simulink model "control_pos_6dof_sinMI"  (R2023b)
settings: Solver=ode45  StartTime=0.0  StopTime=tsim  FixedStep=tstep  MaxStep=tstep  RelTol=tstep/10
undefined symbols (not defined in the file): a0, a1, robot_params, t_qeq_init, t_tr_init, tau_L, tr_ref
(part 5 of 7)

== matlab function control_pos_6dof_sinMI/Controlador/Controlador no lineal ==
  data: robot_params input; tau_R output size=[6,1]; q_ref input size=[6,1]; dq_ref input size=[6,1]; ddq_ref input size=[6,1]; q input size=[6,1]; dq input size=[6,1]; A0 input size=[6,1]; A1 input size=[6,1]
function tau_R = fcn(robot_params,q_ref,dq_ref,ddq_ref,q,dq,A0,A1)

% l1 = robot_params.l(1);
l2 = robot_params.l(2);
l3 = robot_params.l(3);
% l4 = robot_params.l(4);
% l5 = robot_params.l(5);
% l6 = robot_params.l(6);

% lc1 = robot_params.lc(1);
lc2 = robot_params.lc(2);
lc3 = robot_params.lc(3);
% lc4 = robot_params.lc(4);
% lc5 = robot_params.lc(5);
% lc6 = robot_params.lc(6);

d1 = robot_params.d(1);
d2 = robot_params.d(2);
d3 = robot_params.d(3);
d4 = robot_params.d(4);
d5 = robot_params.d(5);
d6 = robot_params.d(6);

% dc1 = robot_params.dc(1);
% dc2 = robot_params.dc(2);
% dc3 = robot_params.dc(3);
dc4 = robot_params.dc(4);
dc5 = robot_params.dc(5);
dc6 = robot_params.dc(6);

m1 = robot_params.m(1);
m2 = robot_params.m(2);
m3 = robot_params.m(3);
m4 = robot_params.m(4);
m5 = robot_params.m(5);
m6 = robot_params.m(6);

g = 9.81;

%Posiciones angulares
q1 = q(1);
q2 = q(2);
q3 = q(3);
q4 = q(4);
q5 = q(5);
q6 = q(6);

%Velocidades angulares
dq1 = dq(1);
dq2 = dq(2);
dq3 = dq(3);
dq4 = dq(4);
dq5 = dq(5);
dq6 = dq(6);

% Matriz de Inercia D
D = zeros(6,6);

D(1,1) = (d1*m1)/2 + (d2*m2)/2 + (d3*m3)/2 + (d4*m4)/2 + (d5*m5)/2 + (d6*m6)/2 + d4^2*m5 + d4^2*m6 + (d5^2*m6)/2 + dc4^2*m4 + (dc5^2*m5)/2 + (3*dc6^2*m6)/4 + (l2^2*m3)/2 + (l2^2*m4)/2 + (l2^2*m5)/2 + (l3^2*m4)/2 + (l2^2*m6)/2 + (l3^2*m5)/2 + (l3^2*m6)/2 + (lc2^2*m2)/2 + (lc3^2*m3)/2 - (dc6^2*m6*cos(2*q2 + 2*q3 + 2*q4 - 2*q5))/8 - (dc6^2*m6*cos(2*q2 + 2*q3 + 2*q4 + 2*q5))/8 - (d5^2*m6*cos(2*q2 + 2*q3 + 2*q4))/2 + (dc6^2*m6*cos(2*q5))/4 - (dc5^2*m5*cos(2*q2 + 2*q3 + 2*q4))/2 + (dc6^2*m6*cos(2*q2 + 2*q3 + 2*q4))/4 + (l2^2*m3*cos(2*q2))/2 + (l2^2*m4*cos(2*q2))/2 + (l2^2*m5*cos(2*q2))/2 + (l2^2*m6*cos(2*q2))/2 + (lc2^2*m2*cos(2*q2))/2 + (l3^2*m4*cos(2*q2 + 2*q3))/2 + (l3^2*m5*cos(2*q2 + 2*q3))/2 + (l3^2*m6*cos(2*q2 + 2*q3))/2 + (lc3^2*m3*cos(2*q2 + 2*q3))/2 + d5*l2*m6*sin(2*q2 + q3 + q4) + dc5*l2*m5*sin(2*q2 + q3 + q4) + (dc6*l2*m6*sin(q3 + q4 - q5))/2 + (d5*dc6*m6*cos(2*q2 + 2*q3 + 2*q4 + q5))/2 + d5*l2*m6*sin(q3 + q4) + dc5*l2*m5*sin(q3 + q4) - (dc6*l3*m6*sin(q4 + q5))/2 + (dc6*l3*m6*sin(2*q2 + 2*q3 + q4 - q5))/2 + 2*d4*dc6*m6*cos(q5) + l2*l3*m4*cos(q3) + l2*l3*m5*cos(q3) + l2*l3*m6*cos(q3) + l2*lc3*m3*cos(q3) + d5*l3*m6*sin(q4) + d5*l3*m6*sin(2*q2 + 2*q3 + q4) + dc5*l3*m5*sin(q4) + dc5*l3*m5*sin(2*q2 + 2*q3 + q4) - (dc6*l2*m6*sin(2*q2 + q3 + q4 + q5))/2 - (d5*dc6*m6*cos(2*q2 + 2*q3 + 2*q4 - q5))/2 + l2*l3*m4*cos(2*q2 + q3) + l2*l3*m5*cos(2*q2 + q3) + l2*l3*m6*cos(2*q2 + q3) + l2*lc3*m3*cos(2*q2 + q3) + (dc6*l3*m6*sin(q4 - q5))/2 - (dc6*l2*m6*sin(q3 + q4 + q5))/2 + (dc6*l2*m6*sin(2*q2 + q3 + q4 - q5))/2 - (dc6*l3*m6*sin(2*q2 + 2*q3 + q4 + q5))/2;
D(1,2) = (dc6^2*m6*cos(q2 + q3 + q4 - 2*q5))/4 - (dc6^2*m6*cos(q2 + q3 + q4 + 2*q5))/4 - (d4*dc6*m6*cos(q2 + q3 + q4 + q5))/2 + (d5*dc6*m6*cos(q2 + q3 + q4 + q5))/2 - (dc6*l3*m6*sin(q2 + q3 - q5))/2 - d4*l3*m5*sin(q2 + q3) - d4*l3*m6*sin(q2 + q3) - dc4*l3*m4*sin(q2 + q3) - (dc6*l2*m6*sin(q2 + q5))/2 + (d4*dc6*m6*cos(q2 + q3 + q4 - q5))/2 + (d5*dc6*m6*cos(q2 + q3 + q4 - q5))/2 - d4*l2*m5*sin(q2) - d4*l2*m6*sin(q2) - dc4*l2*m4*sin(q2) + d4*d5*m6*cos(q2 + q3 + q4) + d4*dc5*m5*cos(q2 + q3 + q4) - (dc6*l2*m6*sin(q2 - q5))/2 - (dc6*l3*m6*sin(q2 + q3 + q5))/2;
D(1,3) = (dc6^2*m6*cos(q2 + q3 + q4 - 2*q5))/4 - (dc6^2*m6*cos(q2 + q3 + q4 + 2*q5))/4 - (d4*dc6*m6*cos(q2 + q3 + q4 + q5))/2 + (d5*dc6*m6*cos(q2 + q3 + q4 + q5))/2 - (dc6*l3*m6*sin(q2 + q3 - q5))/2 - d4*l3*m5*sin(q2 + q3) - d4*l3*m6*sin(q2 + q3) - dc4*l3*m4*sin(q2 + q3) + (d4*dc6*m6*cos(q2 + q3 + q4 - q5))/2 + (d5*dc6*m6*cos(q2 + q3 + q4 - q5))/2 + d4*d5*m6*cos(q2 + q3 + q4) + d4*dc5*m5*cos(q2 + q3 + q4) - (dc6*l3*m6*sin(q2 + q3 + q5))/2;
D(1,4) = (dc6^2*m6*cos(q2 + q3 + q4 - 2*q5))/4 - (dc6^2*m6*cos(q2 + q3 + q4 + 2*q5))/4 - (d4*dc6*m6*cos(q2 + q3 + q4 + q5))/2 + (d5*dc6*m6*cos(q2 + q3 + q4 + q5))/2 + (d4*dc6*m6*cos(q2 + q3 + q4 - q5))/2 + (d5*dc6*m6*cos(q2 + q3 + q4 - q5))/2 + d4*d5*m6*cos(q2 + q3 + q4) + d4*dc5*m5*cos(q2 + q3 + q4);
D(1,5) = -(dc6*m6*(d4*cos(q2 + q3 + q4 + q5) + d5*cos(q2 + q3 + q4 + q5) + l3*sin(q2 + q3 - q5) - l2*sin(q2 + q5) + d4*cos(q2 + q3 + q4 - q5) - d5*cos(q2 + q3 + q4 - q5) + 2*dc6*cos(q2 + q3 + q4) + l2*sin(q2 - q5) - l3*sin(q2 + q3 + q5)))/2;
D(1,6) = 0;

D(2,1) = (dc6^2*m6*cos(q2 + q3 + q4 - 2*q5))/4 - (dc6^2*m6*cos(q2 + q3 + q4 + 2*q5))/4 - (d4*dc6*m6*cos(q2 + q3 + q4 + q5))/2 + (d5*dc6*m6*cos(q2 + q3 + q4 + q5))/2 - (dc6*l3*m6*sin(q2 + q3 - q5))/2 - d4*l3*m5*sin(q2 + q3) - d4*l3*m6*sin(q2 + q3) - dc4*l3*m4*sin(q2 + q3) - (dc6*l2*m6*sin(q2 + q5))/2 + (d4*dc6*m6*cos(q2 + q3 + q4 - q5))/2 + (d5*dc6*m6*cos(q2 + q3 + q4 - q5))/2 - d4*l2*m5*sin(q2) - d4*l2*m6*sin(q2) - dc4*l2*m4*sin(q2) + d4*d5*m6*cos(q2 + q3 + q4) + d4*dc5*m5*cos(q2 + q3 + q4) - (dc6*l2*m6*sin(q2 - q5))/2 - (dc6*l3*m6*sin(q2 + q3 + q5))/2;
D(2,2) = (d2*m2)/2 + (d3*m3)/2 + d4*m4 + (d5*m5)/2 + d5^2*m6 + dc5^2*m5 + (dc6^2*m6)/2 + l2^2*m3 + l2^2*m4 + l2^2*m5 + l3^2*m4 + l2^2*m6 + l3^2*m5 + l3^2*m6 + lc2^2*m2 + lc3^2*m3 - (dc6^2*m6*cos(2*q5))/2 + 2*d5*l2*m6*sin(q3 + q4) + 2*dc5*l2*m5*sin(q3 + q4) + 2*l2*l3*m4*cos(q3) + 2*l2*l3*m5*cos(q3) + 2*l2*l3*m6*cos(q3) + 2*l2*lc3*m3*cos(q3) + 2*d5*l3*m6*sin(q4) + 2*dc5*l3*m5*sin(q4) - 2*dc6*l3*m6*cos(q4)*sin(q5) - 2*dc6*l2*m6*cos(q3)*cos(q4)*sin(q5) + 2*dc6*l2*m6*sin(q3)*sin(q4)*sin(q5);
D(2,3) = d5^2*m6 + dc5^2*m5 + (dc6^2*m6)/2 + l3^2*m4 + l3^2*m5 + l3^2*m6 + lc3^2*m3 - (dc6^2*m6*cos(2*q5))/2 + d5*l2*m6*sin(q3 + q4) + dc5*l2*m5*sin(q3 + q4) + l2*l3*m4*cos(q3) + l2*l3*m5*cos(q3) + l2*l3*m6*cos(q3) + l2*lc3*m3*cos(q3) + 2*d5*l3*m6*sin(q4) + 2*dc5*l3*m5*sin(q4) - 2*dc6*l3*m6*cos(q4)*sin(q5) - dc6*l2*m6*cos(q3)*cos(q4)*sin(q5) + dc6*l2*m6*sin(q3)*sin(q4)*sin(q5);
D(2,4) = d5^2*m6 + dc5^2*m5 + (dc6^2*m6)/2 - (dc6^2*m6*cos(2*q5))/2 + d5*l2*m6*sin(q3 + q4) + dc5*l2*m5*sin(q3 + q4) + d5*l3*m6*sin(q4) + dc5*l3*m5*sin(q4) - dc6*l3*m6*cos(q4)*sin(q5) - dc6*l2*m6*cos(q3)*cos(q4)*sin(q5) + dc6*l2*m6*sin(q3)*sin(q4)*sin(q5);
D(2,5) = -dc6*m6*cos(q5)*(d5 + l2*sin(q3 + q4) + l3*sin(q4));
D(2,6) = 0;

D(3,1) = (dc6^2*m6*cos(q2 + q3 + q4 - 2*q5))/4 - (dc6^2*m6*cos(q2 + q3 + q4 + 2*q5))/4 - (d4*dc6*m6*cos(q2 + q3 + q4 + q5))/2 + (d5*dc6*m6*cos(q2 + q3 + q4 + q5))/2 - (dc6*l3*m6*sin(q2 + q3 - q5))/2 - d4*l3*m5*sin(q2 + q3) - d4*l3*m6*sin(q2 + q3) - dc4*l3*m4*sin(q2 + q3) + (d4*dc6*m6*cos(q2 + q3 + q4 - q5))/2 + (d5*dc6*m6*cos(q2 + q3 + q4 - q5))/2 + d4*d5*m6*cos(q2 + q3 + q4) + d4*dc5*m5*cos(q2 + q3 + q4) - (dc6*l3*m6*sin(q2 + q3 + q5))/2;
D(3,2) = d5^2*m6 + dc5^2*m5 + (dc6^2*m6)/2 + l3^2*m4 + l3^2*m5 + l3^2*m6 + lc3^2*m3 - (dc6^2*m6*cos(2*q5))/2 + d5*l2*m6*sin(q3 + q4) + dc5*l2*m5*sin(q3 + q4) + l2*l3*m4*cos(q3) + l2*l3*m5*cos(q3) + l2*l3*m6*cos(q3) + l2*lc3*m3*cos(q3) + 2*d5*l3*m6*sin(q4) + 2*dc5*l3*m5*sin(q4) - 2*dc6*l3*m6*cos(q4)*sin(q5) - dc6*l2*m6*cos(q3)*cos(q4)*sin(q5) + dc6*l2*m6*sin(q3)*sin(q4)*sin(q5);
D(3,3) = (d3*m3)/2 + d4*m4 + (d5*m5)/2 + d5^2*m6 + dc5^2*m5 + l3^2*m4 + l3^2*m5 + l3^2*m6 + lc3^2*m3 + dc6^2*m6*sin(q5)^2 + 2*d5*l3*m6*sin(q4) + 2*dc5*l3*m5*sin(q4) - 2*dc6*l3*m6*cos(q4)*sin(q5);
D(3,4) = d5^2*m6 + dc5^2*m5 + dc6^2*m6*sin(q5)^2 + d5*l3*m6*sin(q4) + dc5*l3*m5*sin(q4) - dc6*l3*m6*cos(q4)*sin(q5);
D(3,5) = -dc6*m6*cos(q5)*(d5 + l3*sin(q4));
D(3,6) = 0;

D(4,1) = (dc6^2*m6*cos(q2 + q3 + q4 - 2*q5))/4 - (dc6^2*m6*cos(q2 + q3 + q4 + 2*q5))/4 - (d4*dc6*m6*cos(q2 + q3 + q4 + q5))/2 + (d5*dc6*m6*cos(q2 + q3 + q4 + q5))/2 + (d4*dc6*m6*cos(q2 + q3 + q4 - q5))/2 + (d5*dc6*m6*cos(q2 + q3 + q4 - q5))/2 + d4*d5*m6*cos(q2 + q3 + q4) + d4*dc5*m5*cos(q2 + q3 + q4);
D(4,2) = d5^2*m6 + dc5^2*m5 + (dc6^2*m6)/2 - (dc6^2*m6*cos(2*q5))/2 + d5*l2*m6*sin(q3 + q4) + dc5*l2*m5*sin(q3 + q4) + d5*l3*m6*sin(q4) + dc5*l3*m5*sin(q4) - dc6*l3*m6*cos(q4)*sin(q5) - dc6*l2*m6*cos(q3)*cos(q4)*sin(q5) + dc6*l2*m6*sin(q3)*sin(q4)*sin(q5);
D(4,3) = d5^2*m6 + dc5^2*m5 + dc6^2*m6*sin(q5)^2 + d5*l3*m6*sin(q4) + dc5*l3*m5*sin(q4) - dc6*l3*m6*cos(q4)*sin(q5);
D(4,4) = d4*m4 + (d5*m5)/2 + d5^2*m6 + dc5^2*m5 + dc6^2*m6 - dc6^2*m6*cos(q5)^2;
D(4,5) = -d5*dc6*m6*cos(q5);
D(4,6) = 0;

D(5,1) = -(dc6*m6*(d4*cos(q2 + q3 + q4 + q5) + d5*cos(q2 + q3 + q4 + q5) + l3*sin(q2 + q3 - q5) - l2*sin(q2 + q5) + d4*cos(q2 + q3 + q4 - q5) - d5*cos(q2 + q3 + q4 - q5) + 2*dc6*cos(q2 + q3 + q4) + l2*sin(q2 - q5) - l3*sin(q2 + q3 + q5)))/2;
D(5,2) = -dc6*m6*cos(q5)*(d5 + l2*sin(q3 + q4) + l3*sin(q4));
D(5,3) = -dc6*m6*cos(q5)*(d5 + l3*sin(q4));
D(5,4) = -d5*dc6*m6*cos(q5);
D(5,5) = (d4*m4)/2 + (d5*m5)/2 + dc6^2*m6;
D(5,6) = 0;

D(6,1) = 0;
D(6,2) = 0;
D(6,3) = 0;
D(6,4) = 0;
D(6,5) = 0;
D(6,6) = 1;

% Matriz de Coriollis C
C = zeros(6,6);

C(1,1) = 0;
C(1,2) = (dc6^2*dq1*m6*sin(2*q2 + 2*q3 + 2*q4 - 2*q5))/4 + (dc6^2*dq1*m6*sin(2*q2 + 2*q3 + 2*q4 + 2*q5))/4 + d5^2*dq1*m6*sin(2*q2 + 2*q3 + 2*q4) + dc5^2*dq1*m5*sin(2*q2 + 2*q3 + 2*q4) - (dc6^2*dq1*m6*sin(2*q2 + 2*q3 + 2*q4))/2 - dq1*l2^2*m3*sin(2*q2) - dq1*l2^2*m4*sin(2*q2) - dq1*l2^2*m5*sin(2*q2) - dq1*l2^2*m6*sin(2*q2) - dq1*lc2^2*m2*sin(2*q2) - dq1*l3^2*m4*sin(2*q2 + 2*q3) - dq1*l3^2*m5*sin(2*q2 + 2*q3) - dq1*l3^2*m6*sin(2*q2 + 2*q3) - dq1*lc3^2*m3*sin(2*q2 + 2*q3) - (dc6^2*dq2*m6*sin(q2 + q3 + q4 - 2*q5))/4 + (dc6^2*dq2*m6*sin(q2 + q3 + q4 + 2*q5))/4 - (dc6*dq2*l2*m6*cos(q2 - q5))/2 + d5*dc6*dq1*m6*sin(2*q2 + 2*q3 + 2*q4 - q5) - (dc6*dq2*l3*m6*cos(q2 + q3 + q5))/2 - 2*dq1*l2*l3*m4*sin(2*q2 + q3) - 2*dq1*l2*l3*m5*sin(2*q2 + q3) - 2*dq1*l2*l3*m6*sin(2*q2 + q3) - 2*dq1*l2*lc3*m3*sin(2*q2 + q3) - d4*d5*dq2*m6*sin(q2 + q3 + q4) - d4*dc5*dq2*m5*sin(q2 + q3 + q4) + dc6*dq1*l2*m6*cos(2*q2 + q3 + q4 - q5) - dc6*dq1*l3*m6*cos(2*q2 + 2*q3 + q4 + q5) + 2*d5*dq1*l2*m6*cos(2*q2 + q3 + q4) + 2*dc5*dq1*l2*m5*cos(2*q2 + q3 + q4) - (dc6*dq2*l3*m6*cos(q2 + q3 - q5))/2 + (d4*dc6*dq2*m6*sin(q2 + q3 + q4 + q5))/2 - (d5*dc6*dq2*m6*sin(q2 + q3 + q4 + q5))/2 - d4*dq2*l3*m5*cos(q2 + q3) - d4*dq2*l3*m6*cos(q2 + q3) - dc4*dq2*l3*m4*cos(q2 + q3) - (dc6*dq2*l2*m6*cos(q2 + q5))/2 + dc6*dq1*l3*m6*cos(2*q2 + 2*q3 + q4 - q5) - d5*dc6*dq1*m6*sin(2*q2 + 2*q3 + 2*q4 + q5) - d4*dq2*l2*m5*cos(q2) - d4*dq2*l2*m6*cos(q2) + 2*d5*dq1*l3*m6*cos(2*q2 + 2*q3 + q4) - dc4*dq2*l2*m4*cos(q2) + 2*dc5*dq1*l3*m5*cos(2*q2 + 2*q3 + q4) - dc6*dq1*l2*m6*cos(2*q2 + q3 + q4 + q5) - (d4*dc6*dq2*m6*sin(q2 + q3 + q4 - q5))/2 - (d5*dc6*dq2*m6*sin(q2 + q3 + q4 - q5))/2;
C(1,3) = (dc6^2*dq1*m6*sin(2*q2 + 2*q3 + 2*q4 - 2*q5))/4 + (dc6^2*dq1*m6*sin(2*q2 + 2*q3 + 2*q4 + 2*q5))/4 + d5^2*dq1*m6*sin(2*q2 + 2*q3 + 2*q4) + dc5^2*dq1*m5*sin(2*q2 + 2*q3 + 2*q4) - (dc6^2*dq1*m6*sin(2*q2 + 2*q3 + 2*q4))/2 - dq1*l3^2*m4*sin(2*q2 + 2*q3) - dq1*l3^2*m5*sin(2*q2 + 2*q3) - dq1*l3^2*m6*sin(2*q2 + 2*q3) - dq1*lc3^2*m3*sin(2*q2 + 2*q3) - (dc6^2*dq2*m6*sin(q2 + q3 + q4 - 2*q5))/2 + (dc6^2*dq2*m6*sin(q2 + q3 + q4 + 2*q5))/2 - (dc6^2*dq3*m6*sin(q2 + q3 + q4 - 2*q5))/4 + (dc6^2*dq3*m6*sin(q2 + q3 + q4 + 2*q5))/4 + d5*dc6*dq1*m6*sin(2*q2 + 2*q3 + 2*q4 - q5) - (dc6*dq1*l2*m6*cos(q3 + q4 + q5))/2 - dc6*dq2*l3*m6*cos(q2 + q3 + q5) - (dc6*dq3*l3*m6*cos(q2 + q3 + q5))/2 - dq1*l2*l3*m4*sin(2*q2 + q3) - dq1*l2*l3*m5*sin(2*q2 + q3) - dq1*l2*l3*m6*sin(2*q2 + q3) - dq1*l2*lc3*m3*sin(2*q2 + q3) - 2*d4*d5*dq2*m6*sin(q2 + q3 + q4) - d4*d5*dq3*m6*sin(q2 + q3 + q4) - 2*d4*dc5*dq2*m5*sin(q2 + q3 + q4) - d4*dc5*dq3*m5*sin(q2 + q3 + q4) + (dc6*dq1*l2*m6*cos(2*q2 + q3 + q4 - q5))/2 - dc6*dq1*l3*m6*cos(2*q2 + 2*q3 + q4 + q5) + d5*dq1*l2*m6*cos(2*q2 + q3 + q4) + dc5*dq1*l2*m5*cos(2*q2 + q3 + q4) + (dc6*dq1*l2*m6*cos(q3 + q4 - q5))/2 - dc6*dq2*l3*m6*cos(q2 + q3 - q5) - (dc6*dq3*l3*m6*cos(q2 + q3 - q5))/2 + d4*dc6*dq2*m6*sin(q2 + q3 + q4 + q5) + (d4*dc6*dq3*m6*sin(q2 + q3 + q4 + q5))/2 - d5*dc6*dq2*m6*sin(q2 + q3 + q4 + q5) - (d5*dc6*dq3*m6*sin(q2 + q3 + q4 + q5))/2 - 2*d4*dq2*l3*m5*cos(q2 + q3) - 2*d4*dq2*l3*m6*cos(q2 + q3) - d4*dq3*l3*m5*cos(q2 + q3) - d4*dq3*l3*m6*cos(q2 + q3) + d5*dq1*l2*m6*cos(q3 + q4) - 2*dc4*dq2*l3*m4*cos(q2 + q3) - dc4*dq3*l3*m4*cos(q2 + q3) + dc5*dq1*l2*m5*cos(q3 + q4) + dc6*dq1*l3*m6*cos(2*q2 + 2*q3 + q4 - q5) - d5*dc6*dq1*m6*sin(2*q2 + 2*q3 + 2*q4 + q5) + 2*d5*dq1*l3*m6*cos(2*q2 + 2*q3 + q4) + 2*dc5*dq1*l3*m5*cos(2*q2 + 2*q3 + q4) - (dc6*dq1*l2*m6*cos(2*q2 + q3 + q4 + q5))/2 - dq1*l2*l3*m4*sin(q3) - dq1*l2*l3*m5*sin(q3) - dq1*l2*l3*m6*sin(q3) - dq1*l2*lc3*m3*sin(q3) - d4*dc6*dq2*m6*sin(q2 + q3 + q4 - q5) - (d4*dc6*dq3*m6*sin(q2 + q3 + q4 - q5))/2 - d5*dc6*dq2*m6*sin(q2 + q3 + q4 - q5) - (d5*dc6*dq3*m6*sin(q2 + q3 + q4 - q5))/2;
C(1,4) = (dc6^2*dq1*m6*sin(2*q2 + 2*q3 + 2*q4 - 2*q5))/4 + (dc6^2*dq1*m6*sin(2*q2 + 2*q3 + 2*q4 + 2*q5))/4 + d5^2*dq1*m6*sin(2*q2 + 2*q3 + 2*q4) + dc5^2*dq1*m5*sin(2*q2 + 2*q3 + 2*q4) - (dc6^2*dq1*m6*sin(2*q2 + 2*q3 + 2*q4))/2 - (dc6^2*dq2*m6*sin(q2 + q3 + q4 - 2*q5))/2 + (dc6^2*dq2*m6*sin(q2 + q3 + q4 + 2*q5))/2 - (dc6^2*dq3*m6*sin(q2 + q3 + q4 - 2*q5))/2 + (dc6^2*dq3*m6*sin(q2 + q3 + q4 + 2*q5))/2 - (dc6^2*dq4*m6*sin(q2 + q3 + q4 - 2*q5))/4 + (dc6^2*dq4*m6*sin(q2 + q3 + q4 + 2*q5))/4 + (dc6*dq1*l3*m6*cos(q4 - q5))/2 + d5*dc6*dq1*m6*sin(2*q2 + 2*q3 + 2*q4 - q5) - (dc6*dq1*l2*m6*cos(q3 + q4 + q5))/2 - 2*d4*d5*dq2*m6*sin(q2 + q3 + q4) - 2*d4*d5*dq3*m6*sin(q2 + q3 + q4) - d4*d5*dq4*m6*sin(q2 + q3 + q4) - 2*d4*dc5*dq2*m5*sin(q2 + q3 + q4) - 2*d4*dc5*dq3*m5*sin(q2 + q3 + q4) - d4*dc5*dq4*m5*sin(q2 + q3 + q4) + (dc6*dq1*l2*m6*cos(2*q2 + q3 + q4 - q5))/2 - (dc6*dq1*l3*m6*cos(2*q2 + 2*q3 + q4 + q5))/2 + d5*dq1*l2*m6*cos(2*q2 + q3 + q4) + dc5*dq1*l2*m5*cos(2*q2 + q3 + q4) + (dc6*dq1*l2*m6*cos(q3 + q4 - q5))/2 + d4*dc6*dq2*m6*sin(q2 + q3 + q4 + q5) + d4*dc6*dq3*m6*sin(q2 + q3 + q4 + q5) - d5*dc6*dq2*m6*sin(q2 + q3 + q4 + q5) + (d4*dc6*dq4*m6*sin(q2 + q3 + q4 + q5))/2 - d5*dc6*dq3*m6*sin(q2 + q3 + q4 + q5) - (d5*dc6*dq4*m6*sin(q2 + q3 + q4 + q5))/2 + d5*dq1*l2*m6*cos(q3 + q4) + dc5*dq1*l2*m5*cos(q3 + q4) - (dc6*dq1*l3*m6*cos(q4 + q5))/2 + (dc6*dq1*l3*m6*cos(2*q2 + 2*q3 + q4 - q5))/2 - d5*dc6*dq1*m6*sin(2*q2 + 2*q3 + 2*q4 + q5) + d5*dq1*l3*m6*cos(q4) + d5*dq1*l3*m6*cos(2*q2 + 2*q3 + q4) + dc5*dq1*l3*m5*cos(q4) + dc5*dq1*l3*m5*cos(2*q2 + 2*q3 + q4) - (dc6*dq1*l2*m6*cos(2*q2 + q3 + q4 + q5))/2 - d4*dc6*dq2*m6*sin(q2 + q3 + q4 - q5) - d4*dc6*dq3*m6*sin(q2 + q3 + q4 - q5) - d5*dc6*dq2*m6*sin(q2 + q3 + q4 - q5) - (d4*dc6*dq4*m6*sin(q2 + q3 + q4 - q5))/2 - d5*dc6*dq3*m6*sin(q2 + q3 + q4 - q5) - (d5*dc6*dq4*m6*sin(q2 + q3 + q4 - q5))/2;
C(1,5) = (dc6*m6*(4*d4*dq2*sin(q2 + q3 + q4 - q5) - 2*dq1*l2*cos(2*q2 + q3 + q4 + q5) - 8*d4*dq1*sin(q5) + 4*d4*dq3*sin(q2 + q3 + q4 - q5) + 4*d4*dq4*sin(q2 + q3 + q4 - q5) - 2*d4*dq5*sin(q2 + q3 + q4 - q5) + 2*d5*dq5*sin(q2 + q3 + q4 - q5) + 2*dc6*dq2*sin(q2 + q3 + q4 - 2*q5) + 2*dc6*dq2*sin(q2 + q3 + q4 + 2*q5) + 2*dc6*dq3*sin(q2 + q3 + q4 - 2*q5) + 2*dc6*dq3*sin(q2 + q3 + q4 + 2*q5) + 2*dc6*dq4*sin(q2 + q3 + q4 - 2*q5) + 2*dc6*dq4*sin(q2 + q3 + q4 + 2*q5) - 2*dq1*l3*cos(q4 - q5) + 2*dq5*l2*cos(q2 - q5) - 2*d5*dq1*sin(2*q2 + 2*q3 + 2*q4 - q5) - dc6*dq1*sin(2*q2 + 2*q3 + 2*q4 - 2*q5) + dc6*dq1*sin(2*q2 + 2*q3 + 2*q4 + 2*q5) - 2*dq1*l2*cos(q3 + q4 + q5) + 2*dq5*l3*cos(q2 + q3 + q5) + 4*dc6*dq2*sin(q2 + q3 + q4) + 4*dc6*dq3*sin(q2 + q3 + q4) + 4*dc6*dq4*sin(q2 + q3 + q4) - 2*dc6*dq1*sin(2*q5) - 2*dq1*l2*cos(2*q2 + q3 + q4 - q5) - 2*dq1*l3*cos(2*q2 + 2*q3 + q4 + q5) - 2*dq1*l2*cos(q3 + q4 - q5) + 2*dq5*l3*cos(q2 + q3 - q5) + 4*d4*dq2*sin(q2 + q3 + q4 + q5) + 4*d4*dq3*sin(q2 + q3 + q4 + q5) + 4*d4*dq4*sin(q2 + q3 + q4 + q5) + 2*d4*dq5*sin(q2 + q3 + q4 + q5) + 2*d5*dq5*sin(q2 + q3 + q4 + q5) - 2*dq1*l3*cos(q4 + q5) + 2*dq5*l2*cos(q2 + q5) - 2*dq1*l3*cos(2*q2 + 2*q3 + q4 - q5) - 2*d5*dq1*sin(2*q2 + 2*q3 + 2*q4 + q5)))/4;
C(1,6) = 0;

C(2,1) = (dc6^2*dq1*m6*sin(2*q2 + 2*q3 + 2*q4))/4 - (dc6^2*dq1*m6*sin(2*q2 + 2*q3 + 2*q4 + 2*q5))/8 - (d5^2*dq1*m6*sin(2*q2 + 2*q3 + 2*q4))/2 - (dc5^2*dq1*m5*sin(2*q2 + 2*q3 + 2*q4))/2 - (dc6^2*dq1*m6*sin(2*q2 + 2*q3 + 2*q4 - 2*q5))/8 + (dq1*l2^2*m3*sin(2*q2))/2 + (dq1*l2^2*m4*sin(2*q2))/2 + (dq1*l2^2*m5*sin(2*q2))/2 + (dq1*l2^2*m6*sin(2*q2))/2 + (dq1*lc2^2*m2*sin(2*q2))/2 + (dq1*l3^2*m4*sin(2*q2 + 2*q3))/2 + (dq1*l3^2*m5*sin(2*q2 + 2*q3))/2 + (dq1*l3^2*m6*sin(2*q2 + 2*q3))/2 + (dq1*lc3^2*m3*sin(2*q2 + 2*q3))/2 - (d5*dc6*dq1*m6*sin(2*q2 + 2*q3 + 2*q4 - q5))/2 + dq1*l2*l3*m4*sin(2*q2 + q3) + dq1*l2*l3*m5*sin(2*q2 + q3) + dq1*l2*l3*m6*sin(2*q2 + q3) + dq1*l2*lc3*m3*sin(2*q2 + q3) - (dc6*dq1*l2*m6*cos(2*q2 + q3 + q4 - q5))/2 + (dc6*dq1*l3*m6*cos(2*q2 + 2*q3 + q4 + q5))/2 - d5*dq1*l2*m6*cos(2*q2 + q3 + q4) - dc5*dq1*l2*m5*cos(2*q2 + q3 + q4) - (dc6*dq1*l3*m6*cos(2*q2 + 2*q3 + q4 - q5))/2 + (d5*dc6*dq1*m6*sin(2*q2 + 2*q3 + 2*q4 + q5))/2 - d5*dq1*l3*m6*cos(2*q2 + 2*q3 + q4) - dc5*dq1*l3*m5*cos(2*q2 + 2*q3 + q4) + (dc6*dq1*l2*m6*cos(2*q2 + q3 + q4 + q5))/2;
C(2,2) = 0;
C(2,3) = -l2*(2*dq2 + dq3)*(l3*m4*sin(q3) + l3*m5*sin(q3) + l3*m6*sin(q3) + lc3*m3*sin(q3) - d5*m6*cos(q3 + q4) - dc5*m5*cos(q3 + q4) - dc6*m6*cos(q3)*sin(q4)*sin(q5) - dc6*m6*cos(q4)*sin(q3)*sin(q5));
C(2,4) = (dc6*dq4*l3*m6*cos(q4 - q5))/2 + 2*d5*dq2*l2*m6*cos(q3 + q4) + 2*d5*dq3*l2*m6*cos(q3 + q4) + d5*dq4*l2*m6*cos(q3 + q4) + 2*dc5*dq2*l2*m5*cos(q3 + q4) + 2*dc5*dq3*l2*m5*cos(q3 + q4) + dc5*dq4*l2*m5*cos(q3 + q4) - (dc6*dq4*l3*m6*cos(q4 + q5))/2 + 2*d5*dq2*l3*m6*cos(q4) + 2*d5*dq3*l3*m6*cos(q4) + d5*dq4*l3*m6*cos(q4) + 2*dc5*dq2*l3*m5*cos(q4) + 2*dc5*dq3*l3*m5*cos(q4) + dc5*dq4*l3*m5*cos(q4) + 2*dc6*dq2*l3*m6*sin(q4)*sin(q5) + 2*dc6*dq3*l3*m6*sin(q4)*sin(q5) + 2*dc6*dq2*l2*m6*cos(q3)*sin(q4)*sin(q5) + 2*dc6*dq2*l2*m6*cos(q4)*sin(q3)*sin(q5) + 2*dc6*dq3*l2*m6*cos(q3)*sin(q4)*sin(q5) + 2*dc6*dq3*l2*m6*cos(q4)*sin(q3)*sin(q5) + dc6*dq4*l2*m6*cos(q3)*sin(q4)*sin(q5) + dc6*dq4*l2*m6*cos(q4)*sin(q3)*sin(q5);
C(2,5) = -(dc6*m6*(2*dq2*l3*cos(q4 - q5) - 2*d5*dq1*sin(q2 + q3 + q4 - q5) - dc6*dq1*sin(q2 + q3 + q4 - 2*q5) - dc6*dq1*sin(q2 + q3 + q4 + 2*q5) - 2*dq1*l2*cos(q2 - q5) - 2*d5*dq5*sin(q5) + 2*dq3*l3*cos(q4 - q5) + 2*dq4*l3*cos(q4 - q5) - dq5*l3*cos(q4 - q5) + 2*dq1*l3*cos(q2 + q3 + q5) + 2*dq2*l2*cos(q3 + q4 + q5) + 2*dq3*l2*cos(q3 + q4 + q5) + 2*dq4*l2*cos(q3 + q4 + q5) + dq5*l2*cos(q3 + q4 + q5) + 2*dc6*dq1*sin(q2 + q3 + q4) - 2*dc6*dq2*sin(2*q5) - 2*dc6*dq3*sin(2*q5) - 2*dc6*dq4*sin(2*q5) - 2*dq1*l3*cos(q2 + q3 - q5) + 2*dq2*l2*cos(q3 + q4 - q5) + 2*dq3*l2*cos(q3 + q4 - q5) + 2*dq4*l2*cos(q3 + q4 - q5) - dq5*l2*cos(q3 + q4 - q5) + 2*d5*dq1*sin(q2 + q3 + q4 + q5) + 2*dq1*l2*cos(q2 + q5) + 2*dq2*l3*cos(q4 + q5) + 2*dq3*l3*cos(q4 + q5) + 2*dq4*l3*cos(q4 + q5) + dq5*l3*cos(q4 + q5)))/2;
C(2,6) = 0;

C(3,1) = (dc6^2*dq1*m6*sin(2*q2 + 2*q3 + 2*q4))/4 - (dc6^2*dq1*m6*sin(2*q2 + 2*q3 + 2*q4 + 2*q5))/8 - (d5^2*dq1*m6*sin(2*q2 + 2*q3 + 2*q4))/2 - (dc5^2*dq1*m5*sin(2*q2 + 2*q3 + 2*q4))/2 - (dc6^2*dq1*m6*sin(2*q2 + 2*q3 + 2*q4 - 2*q5))/8 + (dq1*l3^2*m4*sin(2*q2 + 2*q3))/2 + (dq1*l3^2*m5*sin(2*q2 + 2*q3))/2 + (dq1*l3^2*m6*sin(2*q2 + 2*q3))/2 + (dq1*lc3^2*m3*sin(2*q2 + 2*q3))/2 - (d5*dc6*dq1*m6*sin(2*q2 + 2*q3 + 2*q4 - q5))/2 + (dc6*dq1*l2*m6*cos(q3 + q4 + q5))/4 + (dq1*l2*l3*m4*sin(2*q2 + q3))/2 + (dq1*l2*l3*m5*sin(2*q2 + q3))/2 + (dq1*l2*l3*m6*sin(2*q2 + q3))/2 + (dq1*l2*lc3*m3*sin(2*q2 + q3))/2 - (dc6*dq1*l2*m6*cos(2*q2 + q3 + q4 - q5))/4 + (dc6*dq1*l3*m6*cos(2*q2 + 2*q3 + q4 + q5))/2 - (d5*dq1*l2*m6*cos(2*q2 + q3 + q4))/2 - (dc5*dq1*l2*m5*cos(2*q2 + q3 + q4))/2 - (dc6*dq1*l2*m6*cos(q3 + q4 - q5))/4 - (d5*dq1*l2*m6*cos(q3 + q4))/2 - (dc5*dq1*l2*m5*cos(q3 + q4))/2 - (dc6*dq1*l3*m6*cos(2*q2 + 2*q3 + q4 - q5))/2 + (d5*dc6*dq1*m6*sin(2*q2 + 2*q3 + 2*q4 + q5))/2 - d5*dq1*l3*m6*cos(2*q2 + 2*q3 + q4) - dc5*dq1*l3*m5*cos(2*q2 + 2*q3 + q4) + (dc6*dq1*l2*m6*cos(2*q2 + q3 + q4 + q5))/4 + (dq1*l2*l3*m4*sin(q3))/2 + (dq1*l2*l3*m5*sin(q3))/2 + (dq1*l2*l3*m6*sin(q3))/2 + (dq1*l2*lc3*m3*sin(q3))/2;
C(3,2) = dq2*l2*(l3*m4*sin(q3) + l3*m5*sin(q3) + l3*m6*sin(q3) + lc3*m3*sin(q3) - d5*m6*cos(q3 + q4) - dc5*m5*cos(q3 + q4) - dc6*m6*cos(q3)*sin(q4)*sin(q5) - dc6*m6*cos(q4)*sin(q3)*sin(q5));
C(3,3) = 0;
C(3,4) = l3*(2*dq2 + 2*dq3 + dq4)*(d5*m6*cos(q4) + dc5*m5*cos(q4) + dc6*m6*sin(q4)*sin(q5));
C(3,5) = -dc6*m6*(dq2*l3*cos(q4 - q5) - d5*dq1*sin(q2 + q3 + q4 - q5) - (dc6*dq1*sin(q2 + q3 + q4 - 2*q5))/2 - (dc6*dq1*sin(q2 + q3 + q4 + 2*q5))/2 - d5*dq5*sin(q5) + dq3*l3*cos(q4 - q5) + dq4*l3*cos(q4 - q5) - (dq5*l3*cos(q4 - q5))/2 + dq1*l3*cos(q2 + q3 + q5) + dc6*dq1*sin(q2 + q3 + q4) - dc6*dq2*sin(2*q5) - dc6*dq3*sin(2*q5) - dc6*dq4*sin(2*q5) - dq1*l3*cos(q2 + q3 - q5) + d5*dq1*sin(q2 + q3 + q4 + q5) + dq2*l3*cos(q4 + q5) + dq3*l3*cos(q4 + q5) + dq4*l3*cos(q4 + q5) + (dq5*l3*cos(q4 + q5))/2);
C(3,6) = 0;

C(4,1) = (dc6^2*dq1*m6*sin(2*q2 + 2*q3 + 2*q4))/4 - (dc6^2*dq1*m6*sin(2*q2 + 2*q3 + 2*q4 + 2*q5))/8 - (d5^2*dq1*m6*sin(2*q2 + 2*q3 + 2*q4))/2 - (dc5^2*dq1*m5*sin(2*q2 + 2*q3 + 2*q4))/2 - (dc6^2*dq1*m6*sin(2*q2 + 2*q3 + 2*q4 - 2*q5))/8 - (dc6*dq1*l3*m6*cos(q4 - q5))/4 - (d5*dc6*dq1*m6*sin(2*q2 + 2*q3 + 2*q4 - q5))/2 + (dc6*dq1*l2*m6*cos(q3 + q4 + q5))/4 - (dc6*dq1*l2*m6*cos(2*q2 + q3 + q4 - q5))/4 + (dc6*dq1*l3*m6*cos(2*q2 + 2*q3 + q4 + q5))/4 - (d5*dq1*l2*m6*cos(2*q2 + q3 + q4))/2 - (dc5*dq1*l2*m5*cos(2*q2 + q3 + q4))/2 - (dc6*dq1*l2*m6*cos(q3 + q4 - q5))/4 - (d5*dq1*l2*m6*cos(q3 + q4))/2 - (dc5*dq1*l2*m5*cos(q3 + q4))/2 + (dc6*dq1*l3*m6*cos(q4 + q5))/4 - (dc6*dq1*l3*m6*cos(2*q2 + 2*q3 + q4 - q5))/4 + (d5*dc6*dq1*m6*sin(2*q2 + 2*q3 + 2*q4 + q5))/2 - (d5*dq1*l3*m6*cos(q4))/2 - (d5*dq1*l3*m6*cos(2*q2 + 2*q3 + q4))/2 - (dc5*dq1*l3*m5*cos(q4))/2 - (dc5*dq1*l3*m5*cos(2*q2 + 2*q3 + q4))/2 + (dc6*dq1*l2*m6*cos(2*q2 + q3 + q4 + q5))/4;
C(4,2) = - dq2*(l2*cos(q3 + q4) + l3*cos(q4))*(d5*m6 + dc5*m5) - dc6*dq2*l3*m6*sin(q4)*sin(q5) - dc6*dq2*l2*m6*cos(q3)*sin(q4)*sin(q5) - dc6*dq2*l2*m6*cos(q4)*sin(q3)*sin(q5);
C(4,3) = -l3*(2*dq2 + dq3)*(d5*m6*cos(q4) + dc5*m5*cos(q4) + dc6*m6*sin(q4)*sin(q5));
C(4,4) = 0;
C(4,5) = (dc6*m6*(2*d5*dq5*sin(q5) + 2*d5*dq1*sin(q2 + q3 + q4 - q5) + dc6*dq1*sin(q2 + q3 + q4 - 2*q5) + dc6*dq1*sin(q2 + q3 + q4 + 2*q5) - 2*dc6*dq1*sin(q2 + q3 + q4) + 2*dc6*dq2*sin(2*q5) + 2*dc6*dq3*sin(2*q5) + 2*dc6*dq4*sin(2*q5) - 2*d5*dq1*sin(q2 + q3 + q4 + q5)))/2;
C(4,6) = 0;

C(5,1) = (dc6*dq1*m6*(2*dc6*sin(2*q5) + 2*l2*cos(2*q2 + q3 + q4 - q5) + 2*l3*cos(2*q2 + 2*q3 + q4 + q5) + 2*l2*cos(q3 + q4 - q5) + 2*l3*cos(q4 + q5) + 2*l3*cos(2*q2 + 2*q3 + q4 - q5) + 2*d5*sin(2*q2 + 2*q3 + 2*q4 + q5) + 8*d4*sin(q5) + 2*l2*cos(2*q2 + q3 + q4 + q5) + 2*l3*cos(q4 - q5) + 2*d5*sin(2*q2 + 2*q3 + 2*q4 - q5) + dc6*sin(2*q2 + 2*q3 + 2*q4 - 2*q5) - dc6*sin(2*q2 + 2*q3 + 2*q4 + 2*q5) + 2*l2*cos(q3 + q4 + q5)))/8;
C(5,2) = (dc6*m6*(dq2*l3*cos(q4 - q5) - dc6*dq1*sin(q2 + q3 + q4 - 2*q5) - dc6*dq1*sin(q2 + q3 + q4 + 2*q5) - 2*dq1*l2*cos(q2 - q5) - 2*d5*dq1*sin(q2 + q3 + q4 - q5) + 2*dq1*l3*cos(q2 + q3 + q5) + dq2*l2*cos(q3 + q4 + q5) + 2*dc6*dq1*sin(q2 + q3 + q4) - dc6*dq2*sin(2*q5) - 2*dq1*l3*cos(q2 + q3 - q5) + dq2*l2*cos(q3 + q4 - q5) + 2*d5*dq1*sin(q2 + q3 + q4 + q5) + 2*dq1*l2*cos(q2 + q5) + dq2*l3*cos(q4 + q5)))/2;
C(5,3) = (dc6*m6*(2*dq2*l3*cos(q4 - q5) - dc6*dq1*sin(q2 + q3 + q4 - 2*q5) - dc6*dq1*sin(q2 + q3 + q4 + 2*q5) - 2*d5*dq1*sin(q2 + q3 + q4 - q5) + dq3*l3*cos(q4 - q5) + 2*dq1*l3*cos(q2 + q3 + q5) + 2*dc6*dq1*sin(q2 + q3 + q4) - 2*dc6*dq2*sin(2*q5) - dc6*dq3*sin(2*q5) - 2*dq1*l3*cos(q2 + q3 - q5) + 2*d5*dq1*sin(q2 + q3 + q4 + q5) + 2*dq2*l3*cos(q4 + q5) + dq3*l3*cos(q4 + q5)))/2;
C(5,4) = -(dc6*m6*(2*d5*dq1*sin(q2 + q3 + q4 - q5) + dc6*dq1*sin(q2 + q3 + q4 - 2*q5) + dc6*dq1*sin(q2 + q3 + q4 + 2*q5) - 2*dc6*dq1*sin(q2 + q3 + q4) + 2*dc6*dq2*sin(2*q5) + 2*dc6*dq3*sin(2*q5) + dc6*dq4*sin(2*q5) - 2*d5*dq1*sin(q2 + q3 + q4 + q5)))/2;
C(5,5) = 0;
C(5,6) = 0;

C(6,1) = 0;
C(6,2) = 0;
C(6,3) = 0;
C(6,4) = 0;
C(6,5) = 0;
C(6,6) = 0;



% Matriz de Gravedad G: 
G = zeros(6,1);

G(1,1) = 0;

G(2,1) = l2*m3*cos(q2) + l2*m4*cos(q2) + l2*m5*cos(q2) + l2*m6*cos(q2) + lc2*m2*cos(q2) + (dc6*m6*sin(q2 + q3 + q4 - q5))/2 + d5*m6*sin(q2 + q3 + q4) + dc5*m5*sin(q2 + q3 + q4) - (dc6*m6*sin(q2 + q3 + q4 + q5))/2 + l3*m4*cos(q2 + q3) + l3*m5*cos(q2 + q3) + l3*m6*cos(q2 + q3) + lc3*m3*cos(q2 + q3);

G(3,1) = (dc6*m6*sin(q2 + q3 + q4 - q5))/2 + d5*m6*sin(q2 + q3 + q4) + dc5*m5*sin(q2 + q3 + q4) - (dc6*m6*sin(q2 + q3 + q4 + q5))/2 + l3*m4*cos(q2 + q3) + l3*m5*cos(q2 + q3) + l3*m6*cos(q2 + q3) + lc3*m3*cos(q2 + q3);

G(4,1) = (dc6*m6*sin(q2 + q3 + q4 - q5))/2 + d5*m6*sin(q2 + q3 + q4) + dc5*m5*sin(q2 + q3 + q4) - (dc6*m6*sin(q2 + q3 + q4 + q5))/2;

G(5,1) = -(dc6*m6*(sin(q2 + q3 + q4 + q5) + sin(q2 + q3 + q4 - q5)))/2;

G(6,1) = 0;


tau_R = D*(ddq_ref+A1.*dq_ref+A0.*q_ref-A1.*dq-A0.*q)+(C*dq+G*g);

== matlab function control_pos_6dof_sinMI/Inicializar posición de robot manipulador/q_init/init_q1/Polinomio 7mo orden q1 ==
  data: t input; q0 input; qpol output; vpol output; apol output; jpol output; q1 input; t0 input; t1 input
function [qpol,vpol,apol,jpol] = fcn(t,q0,q1,t0,t1)


% t,q0,q1,v0,v1,ac0,ac1,j0,j1,t0,t1)
%Trayectoria de referencia

% q0 = 0;
% q1 = 0;

v0 = 0;
v1 = 0;

ac0 = 0;
ac1 = 0;

j0 = 0;
j1 = 0;

% t0 = 0;
% t1 = pi/4;

% Coeficientes de un polinomio de 7mo grado

h = q1 - q0;
T = t1 - t0;

a = zeros(7+1,1);

a(1) = q0;
a(2) = v0;
a(3) = ac0/2;
a(4) = j0/6;
a(5) = (210*h-T*((30*ac0-15*ac1)*T+(4*j0+j1)*T^2+120*v0+90*v1))/(6*T^4);
a(6) = (-168*h-T*((20*ac0-14*ac1)*T+(2*j0+j1)*T^2+90*v0+78*v1))/(2*T^5);
a(7) = (420*h-T*((45*ac0-39*ac1)*T+(4*j0+3*j1)*T^2+216*v0+204*v1))/(6*T^6);
a(8) = (-120*h-T*((12*ac0-12*ac1)*T+(j0+j1)*T^2+60*v0+60*v1))/(6*T^7);

qa = flip(a')';
va = polyder(qa')';
aa = polyder(va')';
ja = polyder(aa')';


if t>=t0 && t<t1
    qpol = polyval(qa,t-t0);
    vpol = polyval(va,t-t0);
    apol = polyval(aa,t-t0);
    jpol = polyval(ja,t-t0);
elseif t>=t1
    qpol = polyval(qa,T);
    vpol = polyval(va,T);
    apol = polyval(aa,T);
    jpol = polyval(ja,T);
else
    qpol = 0;
    vpol = 0;
    apol = 0;
    jpol = 0;
end

== matlab function control_pos_6dof_sinMI/Inicializar posición de robot manipulador/q_init/init_q2/Polinomio 7mo orden q0 ==
  data: t input; q0 input; qpol output; vpol output; apol output; jpol output; q1 input; t0 input; t1 input
function [qpol,vpol,apol,jpol] = fcn(t,q0,q1,t0,t1)


% t,q0,q1,v0,v1,ac0,ac1,j0,j1,t0,t1)
%Trayectoria de referencia

% q0 = 0;
% q1 = 0;

v0 = 0;
v1 = 0;

ac0 = 0;
ac1 = 0;

j0 = 0;
j1 = 0;

% t0 = 0;
% t1 = pi/4;

% Coeficientes de un polinomio de 7mo grado

h = q1 - q0;
T = t1 - t0;

a = zeros(7+1,1);

a(1) = q0;
a(2) = v0;
a(3) = ac0/2;
a(4) = j0/6;
a(5) = (210*h-T*((30*ac0-15*ac1)*T+(4*j0+j1)*T^2+120*v0+90*v1))/(6*T^4);
a(6) = (-168*h-T*((20*ac0-14*ac1)*T+(2*j0+j1)*T^2+90*v0+78*v1))/(2*T^5);
a(7) = (420*h-T*((45*ac0-39*ac1)*T+(4*j0+3*j1)*T^2+216*v0+204*v1))/(6*T^6);
a(8) = (-120*h-T*((12*ac0-12*ac1)*T+(j0+j1)*T^2+60*v0+60*v1))/(6*T^7);

qa = flip(a')';
va = polyder(qa')';
aa = polyder(va')';
ja = polyder(aa')';


if t>=t0 && t<t1
    qpol = polyval(qa,t-t0);
    vpol = polyval(va,t-t0);
    apol = polyval(aa,t-t0);
    jpol = polyval(ja,t-t0);
elseif t>=t1
    qpol = polyval(qa,T);
    vpol = polyval(va,T);
    apol = polyval(aa,T);
    jpol = polyval(ja,T);
else
    qpol = q0;
    vpol = v0;
    apol = ac0;
    jpol = j0;
end

== matlab function control_pos_6dof_sinMI/Inicializar posición de robot manipulador/q_init/init_q2/Polinomio 7mo orden q1 ==
  data: t input; q0 input; qpol output; vpol output; apol output; jpol output; q1 input; t0 input; t1 input
function [qpol,vpol,apol,jpol] = fcn(t,q0,q1,t0,t1)


% t,q0,q1,v0,v1,ac0,ac1,j0,j1,t0,t1)
%Trayectoria de referencia

% q0 = 0;
% q1 = 0;

v0 = 0;
v1 = 0;

ac0 = 0;
ac1 = 0;

j0 = 0;
j1 = 0;

% t0 = 0;
% t1 = pi/4;

% Coeficientes de un polinomio de 7mo grado

h = q1 - q0;
T = t1 - t0;

a = zeros(7+1,1);

a(1) = q0;
a(2) = v0;
a(3) = ac0/2;
a(4) = j0/6;
a(5) = (210*h-T*((30*ac0-15*ac1)*T+(4*j0+j1)*T^2+120*v0+90*v1))/(6*T^4);
a(6) = (-168*h-T*((20*ac0-14*ac1)*T+(2*j0+j1)*T^2+90*v0+78*v1))/(2*T^5);
a(7) = (420*h-T*((45*ac0-39*ac1)*T+(4*j0+3*j1)*T^2+216*v0+204*v1))/(6*T^6);
a(8) = (-120*h-T*((12*ac0-12*ac1)*T+(j0+j1)*T^2+60*v0+60*v1))/(6*T^7);

qa = flip(a')';
va = polyder(qa')';
aa = polyder(va')';
ja = polyder(aa')';


if t>=t0 && t<t1
    qpol = polyval(qa,t-t0);
    vpol = polyval(va,t-t0);
    apol = polyval(aa,t-t0);
    jpol = polyval(ja,t-t0);
elseif t>=t1
    qpol = polyval(qa,T);
    vpol = polyval(va,T);
    apol = polyval(aa,T);
    jpol = polyval(ja,T);
else
    qpol = 0;
    vpol = 0;
    apol = 0;
    jpol = 0;
end

== matlab function control_pos_6dof_sinMI/Inicializar posición de robot manipulador/q_init/init_q3/Polinomio 7mo orden q0 ==
  data: t input; q0 input; qpol output; vpol output; apol output; jpol output; q1 input; t0 input; t1 input
function [qpol,vpol,apol,jpol] = fcn(t,q0,q1,t0,t1)


% t,q0,q1,v0,v1,ac0,ac1,j0,j1,t0,t1)
%Trayectoria de referencia

% q0 = 0;
% q1 = 0;

v0 = 0;
v1 = 0;

ac0 = 0;
ac1 = 0;

j0 = 0;
j1 = 0;

% t0 = 0;
% t1 = pi/4;

% Coeficientes de un polinomio de 7mo grado

h = q1 - q0;
T = t1 - t0;

a = zeros(7+1,1);

a(1) = q0;
a(2) = v0;
a(3) = ac0/2;
a(4) = j0/6;
a(5) = (210*h-T*((30*ac0-15*ac1)*T+(4*j0+j1)*T^2+120*v0+90*v1))/(6*T^4);
a(6) = (-168*h-T*((20*ac0-14*ac1)*T+(2*j0+j1)*T^2+90*v0+78*v1))/(2*T^5);
a(7) = (420*h-T*((45*ac0-39*ac1)*T+(4*j0+3*j1)*T^2+216*v0+204*v1))/(6*T^6);
a(8) = (-120*h-T*((12*ac0-12*ac1)*T+(j0+j1)*T^2+60*v0+60*v1))/(6*T^7);

qa = flip(a')';
va = polyder(qa')';
aa = polyder(va')';
ja = polyder(aa')';


if t>=t0 && t<t1
    qpol = polyval(qa,t-t0);
    vpol = polyval(va,t-t0);
    apol = polyval(aa,t-t0);
    jpol = polyval(ja,t-t0);
elseif t>=t1
    qpol = polyval(qa,T);
    vpol = polyval(va,T);
    apol = polyval(aa,T);
    jpol = polyval(ja,T);
else
    qpol = q0;
    vpol = v0;
    apol = ac0;
    jpol = j0;
end

== matlab function control_pos_6dof_sinMI/Inicializar posición de robot manipulador/q_init/init_q3/Polinomio 7mo orden q1 ==
  data: t input; q0 input; qpol output; vpol output; apol output; jpol output; q1 input; t0 input; t1 input
function [qpol,vpol,apol,jpol] = fcn(t,q0,q1,t0,t1)


% t,q0,q1,v0,v1,ac0,ac1,j0,j1,t0,t1)
%Trayectoria de referencia

% q0 = 0;
% q1 = 0;

v0 = 0;
v1 = 0;

ac0 = 0;
ac1 = 0;

j0 = 0;
j1 = 0;

% t0 = 0;
% t1 = pi/4;

% Coeficientes de un polinomio de 7mo grado

h = q1 - q0;
T = t1 - t0;

a = zeros(7+1,1);

a(1) = q0;
a(2) = v0;
a(3) = ac0/2;
a(4) = j0/6;
a(5) = (210*h-T*((30*ac0-15*ac1)*T+(4*j0+j1)*T^2+120*v0+90*v1))/(6*T^4);
a(6) = (-168*h-T*((20*ac0-14*ac1)*T+(2*j0+j1)*T^2+90*v0+78*v1))/(2*T^5);
a(7) = (420*h-T*((45*ac0-39*ac1)*T+(4*j0+3*j1)*T^2+216*v0+204*v1))/(6*T^6);
a(8) = (-120*h-T*((12*ac0-12*ac1)*T+(j0+j1)*T^2+60*v0+60*v1))/(6*T^7);

qa = flip(a')';
va = polyder(qa')';
aa = polyder(va')';
ja = polyder(aa')';


if t>=t0 && t<t1
    qpol = polyval(qa,t-t0);
    vpol = polyval(va,t-t0);
    apol = polyval(aa,t-t0);
    jpol = polyval(ja,t-t0);
elseif t>=t1
    qpol = polyval(qa,T);
    vpol = polyval(va,T);
    apol = polyval(aa,T);
    jpol = polyval(ja,T);
else
    qpol = 0;
    vpol = 0;
    apol = 0;
    jpol = 0;
end

== matlab function control_pos_6dof_sinMI/Inicializar posición de robot manipulador/q_init/init_q4/Polinomio 7mo orden q0 ==
  data: t input; q0 input; qpol output; vpol output; apol output; jpol output; q1 input; t0 input; t1 input
function [qpol,vpol,apol,jpol] = fcn(t,q0,q1,t0,t1)


% t,q0,q1,v0,v1,ac0,ac1,j0,j1,t0,t1)
%Trayectoria de referencia

% q0 = 0;
% q1 = 0;

v0 = 0;
v1 = 0;

ac0 = 0;
ac1 = 0;

j0 = 0;
j1 = 0;

% t0 = 0;
% t1 = pi/4;

% Coeficientes de un polinomio de 7mo grado

h = q1 - q0;
T = t1 - t0;

a = zeros(7+1,1);

a(1) = q0;
a(2) = v0;
a(3) = ac0/2;
a(4) = j0/6;
a(5) = (210*h-T*((30*ac0-15*ac1)*T+(4*j0+j1)*T^2+120*v0+90*v1))/(6*T^4);
a(6) = (-168*h-T*((20*ac0-14*ac1)*T+(2*j0+j1)*T^2+90*v0+78*v1))/(2*T^5);
a(7) = (420*h-T*((45*ac0-39*ac1)*T+(4*j0+3*j1)*T^2+216*v0+204*v1))/(6*T^6);
a(8) = (-120*h-T*((12*ac0-12*ac1)*T+(j0+j1)*T^2+60*v0+60*v1))/(6*T^7);

qa = flip(a')';
va = polyder(qa')';
aa = polyder(va')';
ja = polyder(aa')';


if t>=t0 && t<t1
    qpol = polyval(qa,t-t0);
    vpol = polyval(va,t-t0);
    apol = polyval(aa,t-t0);
    jpol = polyval(ja,t-t0);
elseif t>=t1
    qpol = polyval(qa,T);
    vpol = polyval(va,T);
    apol = polyval(aa,T);
    jpol = polyval(ja,T);
else
    qpol = q0;
    vpol = v0;
    apol = ac0;
    jpol = j0;
end

== matlab function control_pos_6dof_sinMI/Inicializar posición de robot manipulador/q_init/init_q4/Polinomio 7mo orden q1 ==
  data: t input; q0 input; qpol output; vpol output; apol output; jpol output; q1 input; t0 input; t1 input
function [qpol,vpol,apol,jpol] = fcn(t,q0,q1,t0,t1)


% t,q0,q1,v0,v1,ac0,ac1,j0,j1,t0,t1)
%Trayectoria de referencia

% q0 = 0;
% q1 = 0;

v0 = 0;
v1 = 0;

ac0 = 0;
ac1 = 0;

j0 = 0;
j1 = 0;

% t0 = 0;
% t1 = pi/4;

% Coeficientes de un polinomio de 7mo grado

h = q1 - q0;
T = t1 - t0;

a = zeros(7+1,1);

a(1) = q0;
a(2) = v0;
a(3) = ac0/2;
a(4) = j0/6;
a(5) = (210*h-T*((30*ac0-15*ac1)*T+(4*j0+j1)*T^2+120*v0+90*v1))/(6*T^4);
a(6) = (-168*h-T*((20*ac0-14*ac1)*T+(2*j0+j1)*T^2+90*v0+78*v1))/(2*T^5);
a(7) = (420*h-T*((45*ac0-39*ac1)*T+(4*j0+3*j1)*T^2+216*v0+204*v1))/(6*T^6);
a(8) = (-120*h-T*((12*ac0-12*ac1)*T+(j0+j1)*T^2+60*v0+60*v1))/(6*T^7);

qa = flip(a')';
va = polyder(qa')';
aa = polyder(va')';
ja = polyder(aa')';


if t>=t0 && t<t1
    qpol = polyval(qa,t-t0);
    vpol = polyval(va,t-t0);
    apol = polyval(aa,t-t0);
    jpol = polyval(ja,t-t0);
elseif t>=t1
    qpol = polyval(qa,T);
    vpol = polyval(va,T);
    apol = polyval(aa,T);
    jpol = polyval(ja,T);
else
    qpol = 0;
    vpol = 0;
    apol = 0;
    jpol = 0;
end

== matlab function control_pos_6dof_sinMI/Inicializar posición de robot manipulador/q_init/init_q5/Polinomio 7mo orden q0 ==
  data: t input; q0 input; qpol output; vpol output; apol output; jpol output; q1 input; t0 input; t1 input
function [qpol,vpol,apol,jpol] = fcn(t,q0,q1,t0,t1)


% t,q0,q1,v0,v1,ac0,ac1,j0,j1,t0,t1)
%Trayectoria de referencia

% q0 = 0;
% q1 = 0;

v0 = 0;
v1 = 0;

ac0 = 0;
ac1 = 0;

j0 = 0;
j1 = 0;

% t0 = 0;
% t1 = pi/4;

% Coeficientes de un polinomio de 7mo grado

h = q1 - q0;
T = t1 - t0;

a = zeros(7+1,1);

a(1) = q0;
a(2) = v0;
a(3) = ac0/2;
a(4) = j0/6;
a(5) = (210*h-T*((30*ac0-15*ac1)*T+(4*j0+j1)*T^2+120*v0+90*v1))/(6*T^4);
a(6) = (-168*h-T*((20*ac0-14*ac1)*T+(2*j0+j1)*T^2+90*v0+78*v1))/(2*T^5);
a(7) = (420*h-T*((45*ac0-39*ac1)*T+(4*j0+3*j1)*T^2+216*v0+204*v1))/(6*T^6);
a(8) = (-120*h-T*((12*ac0-12*ac1)*T+(j0+j1)*T^2+60*v0+60*v1))/(6*T^7);

qa = flip(a')';
va = polyder(qa')';
aa = polyder(va')';
ja = polyder(aa')';


if t>=t0 && t<t1
    qpol = polyval(qa,t-t0);
    vpol = polyval(va,t-t0);
    apol = polyval(aa,t-t0);
    jpol = polyval(ja,t-t0);
elseif t>=t1
    qpol = polyval(qa,T);
    vpol = polyval(va,T);
    apol = polyval(aa,T);
    jpol = polyval(ja,T);
else
    qpol = q0;
    vpol = v0;
    apol = ac0;
    jpol = j0;
end

== matlab function control_pos_6dof_sinMI/Inicializar posición de robot manipulador/q_init/init_q5/Polinomio 7mo orden q1 ==
  data: t input; q0 input; qpol output; vpol output; apol output; jpol output; q1 input; t0 input; t1 input
function [qpol,vpol,apol,jpol] = fcn(t,q0,q1,t0,t1)


% t,q0,q1,v0,v1,ac0,ac1,j0,j1,t0,t1)
%Trayectoria de referencia

% q0 = 0;
% q1 = 0;

v0 = 0;
v1 = 0;

ac0 = 0;
ac1 = 0;

j0 = 0;
j1 = 0;

% t0 = 0;
% t1 = pi/4;

% Coeficientes de un polinomio de 7mo grado

h = q1 - q0;
T = t1 - t0;

a = zeros(7+1,1);

a(1) = q0;
a(2) = v0;
a(3) = ac0/2;
a(4) = j0/6;
a(5) = (210*h-T*((30*ac0-15*ac1)*T+(4*j0+j1)*T^2+120*v0+90*v1))/(6*T^4);
a(6) = (-168*h-T*((20*ac0-14*ac1)*T+(2*j0+j1)*T^2+90*v0+78*v1))/(2*T^5);
a(7) = (420*h-T*((45*ac0-39*ac1)*T+(4*j0+3*j1)*T^2+216*v0+204*v1))/(6*T^6);
a(8) = (-120*h-T*((12*ac0-12*ac1)*T+(j0+j1)*T^2+60*v0+60*v1))/(6*T^7);

qa = flip(a')';
va = polyder(qa')';
aa = polyder(va')';
ja = polyder(aa')';


if t>=t0 && t<t1
    qpol = polyval(qa,t-t0);
    vpol = polyval(va,t-t0);
    apol = polyval(aa,t-t0);
    jpol = polyval(ja,t-t0);
elseif t>=t1
    qpol = polyval(qa,T);
    vpol = polyval(va,T);
    apol = polyval(aa,T);
    jpol = polyval(ja,T);
else
    qpol = 0;
    vpol = 0;
    apol = 0;
    jpol = 0;
end

== matlab function control_pos_6dof_sinMI/Inicializar posición de robot manipulador/q_init/init_q6/Polinomio 7mo orden q0 ==
  data: t input; q0 input; qpol output; vpol output; apol output; jpol output; q1 input; t0 input; t1 input
function [qpol,vpol,apol,jpol] = fcn(t,q0,q1,t0,t1)


% t,q0,q1,v0,v1,ac0,ac1,j0,j1,t0,t1)
%Trayectoria de referencia

% q0 = 0;
% q1 = 0;

v0 = 0;
v1 = 0;

ac0 = 0;
ac1 = 0;

j0 = 0;
j1 = 0;

% t0 = 0;
% t1 = pi/4;

% Coeficientes de un polinomio de 7mo grado

h = q1 - q0;
T = t1 - t0;

a = zeros(7+1,1);

a(1) = q0;
a(2) = v0;
a(3) = ac0/2;
a(4) = j0/6;
a(5) = (210*h-T*((30*ac0-15*ac1)*T+(4*j0+j1)*T^2+120*v0+90*v1))/(6*T^4);
a(6) = (-168*h-T*((20*ac0-14*ac1)*T+(2*j0+j1)*T^2+90*v0+78*v1))/(2*T^5);
a(7) = (420*h-T*((45*ac0-39*ac1)*T+(4*j0+3*j1)*T^2+216*v0+204*v1))/(6*T^6);
a(8) = (-120*h-T*((12*ac0-12*ac1)*T+(j0+j1)*T^2+60*v0+60*v1))/(6*T^7);

qa = flip(a')';
va = polyder(qa')';
aa = polyder(va')';
ja = polyder(aa')';


if t>=t0 && t<t1
    qpol = polyval(qa,t-t0);
    vpol = polyval(va,t-t0);
    apol = polyval(aa,t-t0);
    jpol = polyval(ja,t-t0);
elseif t>=t1
    qpol = polyval(qa,T);
    vpol = polyval(va,T);
    apol = polyval(aa,T);
    jpol = polyval(ja,T);
else
    qpol = q0;
    vpol = v0;
    apol = ac0;
    jpol = j0;
end

== matlab function control_pos_6dof_sinMI/Inicializar posición de robot manipulador/dq_init/q2/Polinomio 7mo orden dq ==
  data: t input; q0 input; qpol output; vpol output; apol output; jpol output; q1 input; t0 input; t1 input
function [qpol,vpol,apol,jpol] = fcn(t,q0,q1,t0,t1)


% t,q0,q1,v0,v1,ac0,ac1,j0,j1,t0,t1)
%Trayectoria de referencia

% q0 = 0;
% q1 = 0;

v0 = 0;
v1 = 0;

ac0 = 0;
ac1 = 0;

j0 = 0;
j1 = 0;

% t0 = 0;
% t1 = pi/4;

% Coeficientes de un polinomio de 7mo grado

h = q1 - q0;
T = t1 - t0;

a = zeros(7+1,1);

a(1) = q0;
a(2) = v0;
a(3) = ac0/2;
a(4) = j0/6;
a(5) = (210*h-T*((30*ac0-15*ac1)*T+(4*j0+j1)*T^2+120*v0+90*v1))/(6*T^4);
a(6) = (-168*h-T*((20*ac0-14*ac1)*T+(2*j0+j1)*T^2+90*v0+78*v1))/(2*T^5);
a(7) = (420*h-T*((45*ac0-39*ac1)*T+(4*j0+3*j1)*T^2+216*v0+204*v1))/(6*T^6);
a(8) = (-120*h-T*((12*ac0-12*ac1)*T+(j0+j1)*T^2+60*v0+60*v1))/(6*T^7);

qa = flip(a')';
va = polyder(qa')';
aa = polyder(va')';
ja = polyder(aa')';


if t>=t0 && t<t1
    qpol = polyval(qa,t-t0);
    vpol = polyval(va,t-t0);
    apol = polyval(aa,t-t0);
    jpol = polyval(ja,t-t0);
elseif t>=t1
    qpol = polyval(qa,T);
    vpol = polyval(va,T);
    apol = polyval(aa,T);
    jpol = polyval(ja,T);
else
    qpol = q0;
    vpol = v0;
    apol = ac0;
    jpol = j0;
end

== matlab function control_pos_6dof_sinMI/Inicializar posición de robot manipulador/q_init/init_q6/Polinomio 7mo orden q1 ==
  data: t input; q0 input; qpol output; vpol output; apol output; jpol output; q1 input; t0 input; t1 input
function [qpol,vpol,apol,jpol] = fcn(t,q0,q1,t0,t1)


% t,q0,q1,v0,v1,ac0,ac1,j0,j1,t0,t1)
%Trayectoria de referencia

% q0 = 0;
% q1 = 0;

v0 = 0;
v1 = 0;

ac0 = 0;
ac1 = 0;

j0 = 0;
j1 = 0;

% t0 = 0;
% t1 = pi/4;

% Coeficientes de un polinomio de 7mo grado

h = q1 - q0;
T = t1 - t0;

a = zeros(7+1,1);

a(1) = q0;
a(2) = v0;
a(3) = ac0/2;
a(4) = j0/6;
a(5) = (210*h-T*((30*ac0-15*ac1)*T+(4*j0+j1)*T^2+120*v0+90*v1))/(6*T^4);
a(6) = (-168*h-T*((20*ac0-14*ac1)*T+(2*j0+j1)*T^2+90*v0+78*v1))/(2*T^5);
a(7) = (420*h-T*((45*ac0-39*ac1)*T+(4*j0+3*j1)*T^2+216*v0+204*v1))/(6*T^6);
a(8) = (-120*h-T*((12*ac0-12*ac1)*T+(j0+j1)*T^2+60*v0+60*v1))/(6*T^7);

qa = flip(a')';
va = polyder(qa')';
aa = polyder(va')';
ja = polyder(aa')';


if t>=t0 && t<t1
    qpol = polyval(qa,t-t0);
    vpol = polyval(va,t-t0);
    apol = polyval(aa,t-t0);
    jpol = polyval(ja,t-t0);
elseif t>=t1
    qpol = polyval(qa,T);
    vpol = polyval(va,T);
    apol = polyval(aa,T);
    jpol = polyval(ja,T);
else
    qpol = 0;
    vpol = 0;
    apol = 0;
    jpol = 0;
end

== matlab function control_pos_6dof_sinMI/Inicializar posición de robot manipulador/dq_init/q6/Polinomio 7mo orden dq ==
  data: t input; q0 input; qpol output; vpol output; apol output; jpol output; q1 input; t0 input; t1 input
function [qpol,vpol,apol,jpol] = fcn(t,q0,q1,t0,t1)


% t,q0,q1,v0,v1,ac0,ac1,j0,j1,t0,t1)
%Trayectoria de referencia

% q0 = 0;
% q1 = 0;

v0 = 0;
v1 = 0;

ac0 = 0;
ac1 = 0;

j0 = 0;
j1 = 0;

% t0 = 0;
% t1 = pi/4;

% Coeficientes de un polinomio de 7mo grado

h = q1 - q0;
T = t1 - t0;

a = zeros(7+1,1);

a(1) = q0;
a(2) = v0;
a(3) = ac0/2;
a(4) = j0/6;
a(5) = (210*h-T*((30*ac0-15*ac1)*T+(4*j0+j1)*T^2+120*v0+90*v1))/(6*T^4);
a(6) = (-168*h-T*((20*ac0-14*ac1)*T+(2*j0+j1)*T^2+90*v0+78*v1))/(2*T^5);
a(7) = (420*h-T*((45*ac0-39*ac1)*T+(4*j0+3*j1)*T^2+216*v0+204*v1))/(6*T^6);
a(8) = (-120*h-T*((12*ac0-12*ac1)*T+(j0+j1)*T^2+60*v0+60*v1))/(6*T^7);

qa = flip(a')';
va = polyder(qa')';
aa = polyder(va')';
ja = polyder(aa')';


if t>=t0 && t<t1
    qpol = polyval(qa,t-t0);
    vpol = polyval(va,t-t0);
    apol = polyval(aa,t-t0);
    jpol = polyval(ja,t-t0);
elseif t>=t1
    qpol = polyval(qa,T);
    vpol = polyval(va,T);
    apol = polyval(aa,T);
    jpol = polyval(ja,T);
else
    qpol = q0;
    vpol = v0;
    apol = ac0;
    jpol = j0;
end

== matlab function control_pos_6dof_sinMI/Inicializar posición de robot manipulador/MATLAB Function ==
  data: t input size=1; qi output size=[6,1]; t_init input size=1; q input size=[6,1]; q_init input
function qi  = fcn(t,t_init,q,q_init)

% qi = q;
if t <= t_init
    qi = q;
else
    qi = q_init;
end

== matlab function control_pos_6dof_sinMI/Inicializar posición de robot manipulador/dq_init1/q4/Polinomio 7mo orden dq ==
  data: t input; q0 input; qpol output; vpol output; apol output; jpol output; q1 input; t0 input; t1 input
function [qpol,vpol,apol,jpol] = fcn(t,q0,q1,t0,t1)


% t,q0,q1,v0,v1,ac0,ac1,j0,j1,t0,t1)
%Trayectoria de referencia

% q0 = 0;
% q1 = 0;

v0 = 0;
v1 = 0;

ac0 = 0;
ac1 = 0;

j0 = 0;
j1 = 0;

% t0 = 0;
% t1 = pi/4;

% Coeficientes de un polinomio de 7mo grado

h = q1 - q0;
T = t1 - t0;

a = zeros(7+1,1);

a(1) = q0;
a(2) = v0;
a(3) = ac0/2;
a(4) = j0/6;
a(5) = (210*h-T*((30*ac0-15*ac1)*T+(4*j0+j1)*T^2+120*v0+90*v1))/(6*T^4);
a(6) = (-168*h-T*((20*ac0-14*ac1)*T+(2*j0+j1)*T^2+90*v0+78*v1))/(2*T^5);
a(7) = (420*h-T*((45*ac0-39*ac1)*T+(4*j0+3*j1)*T^2+216*v0+204*v1))/(6*T^6);
a(8) = (-120*h-T*((12*ac0-12*ac1)*T+(j0+j1)*T^2+60*v0+60*v1))/(6*T^7);

qa = flip(a')';
va = polyder(qa')';
aa = polyder(va')';
ja = polyder(aa')';


if t>=t0 && t<t1
    qpol = polyval(qa,t-t0);
    vpol = polyval(va,t-t0);
    apol = polyval(aa,t-t0);
    jpol = polyval(ja,t-t0);
elseif t>=t1
    qpol = polyval(qa,T);
    vpol = polyval(va,T);
    apol = polyval(aa,T);
    jpol = polyval(ja,T);
else
    qpol = q0;
    vpol = v0;
    apol = ac0;
    jpol = j0;
end

== matlab function control_pos_6dof_sinMI/Inicializar posición de robot manipulador/dq_init1/q5/Polinomio 7mo orden dq ==
  data: t input; q0 input; qpol output; vpol output; apol output; jpol output; q1 input; t0 input; t1 input
function [qpol,vpol,apol,jpol] = fcn(t,q0,q1,t0,t1)


% t,q0,q1,v0,v1,ac0,ac1,j0,j1,t0,t1)
%Trayectoria de referencia

% q0 = 0;
% q1 = 0;

v0 = 0;
v1 = 0;

ac0 = 0;
ac1 = 0;

j0 = 0;
j1 = 0;

% t0 = 0;
% t1 = pi/4;

% Coeficientes de un polinomio de 7mo grado

h = q1 - q0;
T = t1 - t0;

a = zeros(7+1,1);

a(1) = q0;
a(2) = v0;
a(3) = ac0/2;
a(4) = j0/6;
a(5) = (210*h-T*((30*ac0-15*ac1)*T+(4*j0+j1)*T^2+120*v0+90*v1))/(6*T^4);
a(6) = (-168*h-T*((20*ac0-14*ac1)*T+(2*j0+j1)*T^2+90*v0+78*v1))/(2*T^5);
a(7) = (420*h-T*((45*ac0-39*ac1)*T+(4*j0+3*j1)*T^2+216*v0+204*v1))/(6*T^6);
a(8) = (-120*h-T*((12*ac0-12*ac1)*T+(j0+j1)*T^2+60*v0+60*v1))/(6*T^7);

qa = flip(a')';
va = polyder(qa')';
aa = polyder(va')';
ja = polyder(aa')';


if t>=t0 && t<t1
    qpol = polyval(qa,t-t0);
    vpol = polyval(va,t-t0);
    apol = polyval(aa,t-t0);
    jpol = polyval(ja,t-t0);
elseif t>=t1
    qpol = polyval(qa,T);
    vpol = polyval(va,T);
    apol = polyval(aa,T);
    jpol = polyval(ja,T);
else
    qpol = q0;
    vpol = v0;
    apol = ac0;
    jpol = j0;
end

== matlab function control_pos_6dof_sinMI/Inicializar posición de robot manipulador/dq_init1/q6/Polinomio 7mo orden dq ==
  data: t input; q0 input; qpol output; vpol output; apol output; jpol output; q1 input; t0 input; t1 input
function [qpol,vpol,apol,jpol] = fcn(t,q0,q1,t0,t1)


% t,q0,q1,v0,v1,ac0,ac1,j0,j1,t0,t1)
%Trayectoria de referencia

% q0 = 0;
% q1 = 0;

v0 = 0;
v1 = 0;

ac0 = 0;
ac1 = 0;

j0 = 0;
j1 = 0;

% t0 = 0;
% t1 = pi/4;

% Coeficientes de un polinomio de 7mo grado

h = q1 - q0;
T = t1 - t0;

a = zeros(7+1,1);

a(1) = q0;
a(2) = v0;
a(3) = ac0/2;
a(4) = j0/6;
a(5) = (210*h-T*((30*ac0-15*ac1)*T+(4*j0+j1)*T^2+120*v0+90*v1))/(6*T^4);
a(6) = (-168*h-T*((20*ac0-14*ac1)*T+(2*j0+j1)*T^2+90*v0+78*v1))/(2*T^5);
a(7) = (420*h-T*((45*ac0-39*ac1)*T+(4*j0+3*j1)*T^2+216*v0+204*v1))/(6*T^6);
a(8) = (-120*h-T*((12*ac0-12*ac1)*T+(j0+j1)*T^2+60*v0+60*v1))/(6*T^7);

qa = flip(a')';
va = polyder(qa')';
aa = polyder(va')';
ja = polyder(aa')';


if t>=t0 && t<t1
    qpol = polyval(qa,t-t0);
    vpol = polyval(va,t-t0);
    apol = polyval(aa,t-t0);
    jpol = polyval(ja,t-t0);
elseif t>=t1
    qpol = polyval(qa,T);
    vpol = polyval(va,T);
    apol = polyval(aa,T);
    jpol = polyval(ja,T);
else
    qpol = q0;
    vpol = v0;
    apol = ac0;
    jpol = j0;
end

== matlab function control_pos_6dof_sinMI/Dinámica inversa (referencia)/Dinámica inversa ==
  data: robot_din input; dq input size=[6,1]; tau_s output size=[6,1]; ddq input size=[6,1]
function tau_s = fcn(robot_din,dq,ddq)

D = robot_din.D;
C = robot_din.C;
G = robot_din.G;
g = robot_din.g;

tau_s = D*ddq + C*dq + G*g;
